simulink model "Example_4_Closed"  (Simulink 8.3)
settings: Solver=ode45  StartTime=0.0  StopTime=40  RelTol=1e-3
settings Model: Creator=Li Jinghao  LastModifiedBy=Li Jinghao
settings DataIOCC: SignalLoggingSaveFormat=Dataset  InspectSignalLogs=on
settings DebuggingCC: UnderspecifiedInitializationDetection=Simplified  StateNameClashWarn=none
settings GRTTargetCC: CombineOutputUpdateFcns=on  GRTInterface=off

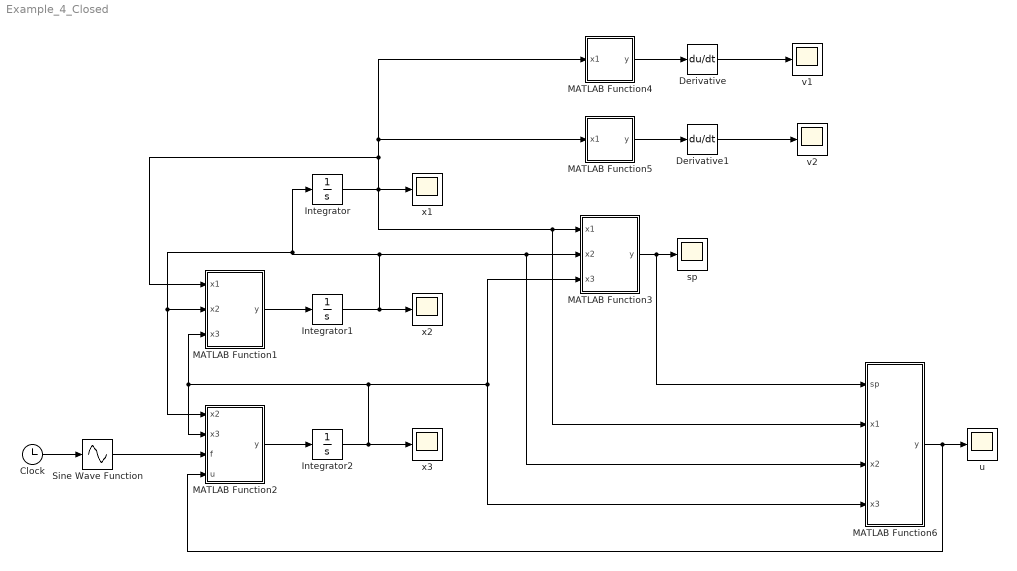
== system Example_4_Closed ==
  Clock : Clock
  Derivative : Derivative
  Derivative1 : Derivative
  Integrator : Integrator  InitialCondition=pi/8
  Integrator1 : Integrator
  Integrator2 : Integrator  InitialCondition=0.8
  MATLAB Function1 : MATLAB Function  TreatAsAtomicUnit=on
  MATLAB Function2 : MATLAB Function  TreatAsAtomicUnit=on
  MATLAB Function3 : MATLAB Function  TreatAsAtomicUnit=on
  MATLAB Function4 : MATLAB Function  TreatAsAtomicUnit=on
  MATLAB Function5 : MATLAB Function  TreatAsAtomicUnit=on
  MATLAB Function6 : MATLAB Function  TreatAsAtomicUnit=on
  Sine Wave Function : Sin  TimeSource=Use external signal  Bias=1  SampleTime=0
  sp : Scope
      settings: TimeRange=40  YMin=-0.2  YMax=1.2  SaveName=s
  u : Scope
      settings: TimeRange=40  SaveName=u
  v1 : Scope
      settings: SaveName=v1
  v2 : Scope
      settings: SaveName=v2
  x1 : Scope
      settings: SaveName=x1
  x2 : Scope
      settings: SaveName=x2
  x3 : Scope
      settings: TimeRange=40  YMin=-0.5  YMax=3  SaveName=x3
  wires:
  Integrator2/1 -> MATLAB Function6/4(x3), MATLAB Function3/3(x3), MATLAB Function2/2(x3), MATLAB Function1/3(x3), x3/1
  Integrator1/1 -> Integrator/1, MATLAB Function2/1(x2), MATLAB Function1/2(x2), MATLAB Function6/3(x2), MATLAB Function3/2(x2), x2/1
  Integrator/1 -> MATLAB Function6/2(x1), MATLAB Function3/1(x1), MATLAB Function4/1(x1), MATLAB Function5/1(x1), MATLAB Function1/1(x1), x1/1
  MATLAB Function1/1(y) -> Integrator1/1
  MATLAB Function2/1(y) -> Integrator2/1
  Clock/1 -> Sine Wave Function/1
  Sine Wave Function/1 -> MATLAB Function2/3(f)
  MATLAB Function3/1(y) -> MATLAB Function6/1(sp), sp/1
  MATLAB Function4/1(y) -> Derivative/1
  MATLAB Function5/1(y) -> Derivative1/1
  MATLAB Function6/1(y) -> MATLAB Function2/4(u), u/1
  Derivative/1 -> v1/1
  Derivative1/1 -> v2/1

== matlab function MATLAB Function1 ==
  data: x1 input double; y output double; x2 input double; x3 input double
function y = fcn(x1,x2,x3)
%#codegen

Jm=0.126*10^-3;
alpha=0.001;
l=0.2;
m=0.1;
km=0.0446;
g=9.81;

y = 1/(Jm+m*l*l)*(-m*g*l*sin(x1)-alpha*x2+km*x3);

== matlab function MATLAB Function3 ==
  data: x1 input double; y output double; x2 input double; x3 input double
function y = fcn(x1,x2,x3)
%#codegen

v1=(2*pi*sin(x1)-3*sqrt(3)*x1)/((2*pi-3*sqrt(3))*x1);
v2=1-v1;
Sp1=[0.5601    1.0593];
Sp2=[1.3211    1.0593];

y=(v1*Sp1+v2*Sp2)*[x1;x2]+x3;

== matlab function MATLAB Function2 ==
  data: x2 input double; y output double; x3 input double; f input double; u input double
function y = fcn(x2,x3,f,u)
%#codegen

R=0.1;
L=92;
ke=0.076;

y = 1/L*(-ke*x2-R*x3+f+u);

== matlab function MATLAB Function4 ==
  data: x1 input double; y output double
function y = fcn(x1)
%#codegen

y=(2*pi*sin(x1)-3*sqrt(3)*x1)/((2*pi-3*sqrt(3))*x1);

== matlab function MATLAB Function5 ==
  data: x1 input double; y output double
function y = fcn(x1)
%#codegen

y=1-(2*pi*sin(x1)-3*sqrt(3)*x1)/((2*pi-3*sqrt(3))*x1);

== matlab function MATLAB Function6 ==
  data: sp input double; x1 input double; y output double; x2 input double; x3 input double
function y = fcn(sp,x1,x2,x3)
%#codegen

v1=(2*pi*sin(x1)-3*sqrt(3)*x1)/((2*pi-3*sqrt(3))*x1);
v2=1-v1;
Sp1=[0.5601    1.0593];
Sp2=[1.3211    1.0593];
A11=[0 1;-47.5521 -0.2424];
A21 =[0 1;-39.3253 -0.2424];
A12=[0;10.8095];
A22=[0;10.8095];
A13=10^-3*[0 -0.8261];
A23=10^-3*[0 -0.8261];
A14=-0.0011;
A24=-0.0011;
B1=0.0109;
kappap=7;
bx1=0.4;
psi1=0.6;
psi2=0.6;
bf=2;
rho1=0.001;
rho=norm(B1)*bf+(psi1*norm(Sp1)+psi2*norm(Sp2))*bx1+rho1;

Sp=v1*Sp1+v2*Sp2;
A1=v1*A11+v2*A21;
A2=v1*A12+v2*A22;
A3=v1*A13+v2*A23;
A4=v1*A14+v2*A24;

y = -inv(B1)*((Sp*A1+A3+kappap*Sp)*[x1;x2]+(Sp*A2+A4+kappap)*x3+rho*sp/norm(sp));
